simulink model "TestLinearisationSystem"  (R2018b)
settings: Solver=VariableStepAuto  StartTime=0.0  StopTime=5  MaxStep=1e-3  RelTol=1e-3
undefined symbols (not defined in the file): kM, m, tauM
libraries: simulink x1
settings Model: Creator=jban039  LastModifiedBy=jban039
settings DataIOCC: InitialState=getstatestruct(op)  LoadInitialState=on

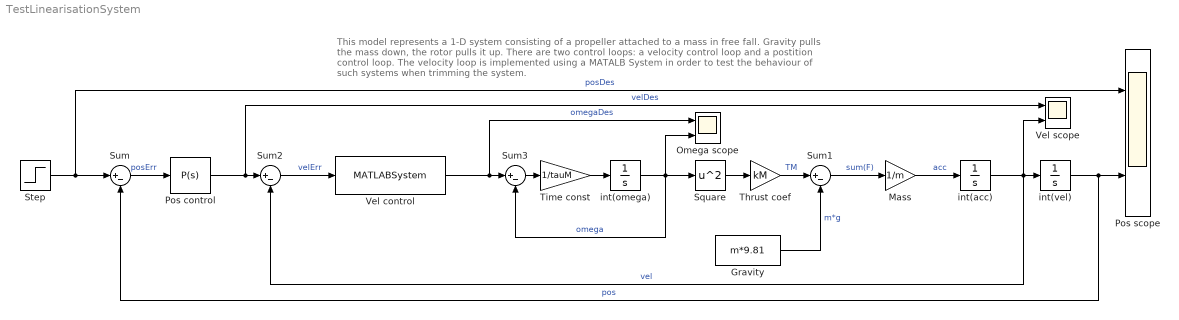
== system TestLinearisationSystem ==
  note: This model represents a 1-D system consisting of a propeller attached to a mass in free fall. Gravity pulls the mass down, the rotor pulls it up.
      | There are two control loops: a velocity control loop and a postition control loop. The velocity loop is implemented using a MATALB System in
      | order to test the behaviour of such systems when trimming the system.
  Gravity : Constant  Value=m*9.81
  Mass : Gain  Gain=1/m
  Omega scope : Scope  NumInputPorts=2
  Pos control : simulink/Continuous/PID Controller  Controller=P  Form=Parallel  TimeDomain=Continuous-time  SampleTime=-1  IntegratorMethod=Forward Euler  FilterMethod=Forward Euler  ControllerParametersSource=internal  P=1.897479840545  I=0  D=0  UseFilter=on  N=100  TunerSelectOption=Transfer Function Based (PID Tuner App)  InitialConditionSource=internal  InitialConditionForIntegrator=0  InitialConditionForFilter=0  DifferentiatorICPrevScaledInput=0  ExternalReset=none  TrackingMode=off  Kt=1  LimitOutput=off  UpperSaturationLimit=inf  LowerSaturationLimit=-inf  LinearizeAsGain=on  AntiWindupMode=none  Kb=1  POutMin=[]  POutMax=[]  IOutMin=[]  IOutMax=[]  DOutMin=[]  DOutMax=[]  NOutMin=[]  NOutMax=[]  SumOutMin=[]  SumOutMax=[]  SaturationOutMin=[]  SaturationOutMax=[]  PParamMin=[]  PParamMax=[]  IParamMin=[]  IParamMax=[]  DParamMin=[]  DParamMax=[]  NParamMin=[]  NParamMax=[]  KbParamMin=[]  KbParamMax=[]  KtParamMin=[]  KtParamMax=[]  KbOutMin=[]  KbOutMax=[]  KtOutMin=[]  KtOutMax=[]  IntegratorOutMin=[]  IntegratorOutMax=[]  FilterOutMin=[]  FilterOutMax=[]  SumI1OutMin=[]  SumI1OutMax=[]  SumI2OutMin=[]  SumI2OutMax=[]  SumI3OutMin=[]  SumI3OutMax=[]  SumI4OutMin=[]  SumI4OutMax=[]  SumDOutMin=[]  SumDOutMax=[]  DifferentiatorOutMin=[]  DifferentiatorOutMax=[]  FilterDiffOutCoefMin=[]  FilterDiffOutCoefMax=[]  ReciprocalOutMin=[]  ReciprocalOutMax=[]  SumDenOutMin=[]  SumDenOutMax=[]  SumNumOutMin=[]  SumNumOutMax=[]  DivideOutMin=[]  DivideOutMax=[]  IntegratorContinuousStateAttributes=''  IntegratorStateMustResolveToSignalObject=off  IntegratorRTWStateStorageClass=Auto  FilterContinuousStateAttributes=''  FilterStateMustResolveToSignalObject=off  FilterRTWStateStorageClass=Auto  ParallelPVariant=InternalParameters  IdealPVariant=Disabled  IVariant=Disabled  DVariant=Disabled  IntegratorVariant=Disabled  SatVariant=Disabled  AWVariant=Disabled  PCopyVariant=Disabled  TRVariant=Disabled  FdbkBlocksVariant=Forward  IdealPFdbkVariant=Disabled  SatFdbkVariant=Disabled  DerivativeFilterVariant=Disabled  NVariant=Disabled  NCopyVariant=Disabled_SignalSpec  FilterICVariant=Disabled  IntegratorICVariant=Disabled  ExternalResetVariant=Disabled  TRSumVariant=Passthrough  SumFdbkVariant=Disabled  SumVariant=Passthrough_P
  Pos scope : Scope  NumInputPorts=2
  Square : Math  Operator=square  SaturateOnIntegerOverflow=on
  Step : Step  SampleTime=0
  Sum{,1..3} (4 alike) : Sum  Inputs=|+-
  Thrust coef : Gain  Gain=kM
  Time const : Gain  Gain=1/tauM
  Vel control : MATLABSystem  System=TestMatlabSystem  Ts=0.005  Kp=0.2  Ki=0.02  SimulateUsing=Code generation
      mask Type: TestMatlabSystem
      mask Display:
      | disp('TestMatlabSystem');
      | port_label('input',1,'u');
      | port_label('output',1,'y');
  Vel scope : Scope  NumInputPorts=2
  int(acc) : Integrator  ContinuousStateAttributes='velocity'
  int(omega) : Integrator  ContinuousStateAttributes='omega'
  int(vel) : Integrator  ContinuousStateAttributes='position'
  wires:
  Step/1 -> Sum/1, Pos scope/1  "posDes"
  int(omega)/1 -> Sum3/2, Omega scope/2, Square/1  "omega"
  Square/1 -> Thrust coef/1
  Thrust coef/1 -> Sum1/1  "TM"
  Gravity/1 -> Sum1/2  "m*g"
  Sum1/1 -> Mass/1  "sum(F)"
  Mass/1 -> int(acc)/1  "acc"
  int(acc)/1 -> Vel scope/2, Sum2/2, int(vel)/1  "vel"
  int(vel)/1 -> Pos scope/2, Sum/2  "pos"
  Sum/1 -> Pos control/1  "posErr"
  Pos control/1 -> Sum2/1, Vel scope/1  "velDes"
  Sum2/1 -> Vel control/1  "velErr"
  Vel control/1 -> Sum3/1, Omega scope/1  "omegaDes"
  Sum3/1 -> Time const/1
  Time const/1 -> int(omega)/1
